simulink model "CH7_4C"  (R2021b)
settings: Solver=ode45  StartTime=0.0  StopTime=4  RelTol=1e-3  EnableMultiTasking=on
libraries: dsparch4 x2
settings Model: Creator=xnote  LastModifiedBy=82102
settings SolverCC: AlgebraicLoopSolver=TrustRegion
settings DataIOCC: LimitDataPoints=on  SaveFormat=Array  SignalLoggingSaveFormat=ModelDataLogs  ReturnWorkspaceOutputs=off
settings OptimizationCC: ExpressionDepthLimit=2147483647  LifeSpan=inf
settings DebuggingCC: UnderspecifiedInitializationDetection=Classic  MergeDetectMultiDrivingBlocksExec=none  SolverPrmCheckMsg=warning  FcnCallInpInsideContextMsg=warning  StateNameClashWarn=warning  SFUnexpectedBacktrackingDiag=warning  SFNoUnconditionalDefaultTransitionDiag=warning  SFExecutionAtInitializationDiag=none  SFMachineParentedDataDiag=warning  ArithmeticOperatorsInVariantConditions=warning
settings HardwareCC: ProdBitPerPointer=32  ProdBitPerSizeT=32  ProdBitPerPtrDiffT=32  ProdLargestAtomicFloat=None  ProdIntDivRoundTo=Undefined  ProdEndianess=Unspecified  ProdWordSize=32  ProdHWDeviceType=32-bit Generic
settings ModelReferenceCC: PropagateSignalLabelsOutOfModel=off
settings SFSimCC: SimUseLocalCustomCode=off  CustomCodeUndefinedFunction=UseInterfaceOnly
settings RTWCC: RTWUseLocalCustomCode=off
settings CodeAppCC: StateflowObjectComments=on
settings GRTTargetCC: TargetLangStandard=C89/C90 (ANSI)  CombineOutputUpdateFcns=off  GRTInterface=on
settings ConfigComp: CovMetricSettings=dw  CovSaveCumulativeToWorkspaceVar=on  CovSaveSingleToWorkspaceVar=on  CovExternalEMLEnable=off

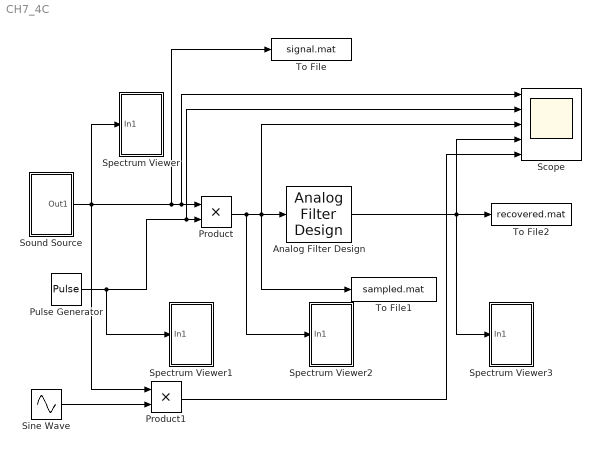
== system CH7_4C ==
  Analog Filter Design : dsparch4/Analog Filter Design  method=Butterworth  filttype=Bandpass  N=8  Wlo=800*pi  Whi=8000*pi  Rp=2  Rs=40
  Product : Product  RndMeth=Zero  SampleTime=1/(16e4)
  Product1 : Product  RndMeth=Zero  SampleTime=1/(16e4)
  Pulse Generator : DiscretePulseGenerator  PulseType=Time based  Period=1/(8e3)  PulseWidth=10
  Scope : Scope  NumInputPorts=5
  Sine Wave : Sin  SampleTime=0
  Sound Source : Subsystem
  Spectrum Viewer : Subsystem
  Spectrum Viewer1 : Subsystem
  Spectrum Viewer2 : Subsystem
  Spectrum Viewer3 : Subsystem
  To File : ToFile  Filename=signal.mat  SampleTime=1/8192
  To File1 : ToFile  Filename=sampled.mat  SampleTime=1/8192
  To File2 : ToFile  Filename=recovered.mat  SampleTime=1/8192
  wires:
  Sound Source/1(Out1) -> Spectrum Viewer/1(In1), To File/1, Product/1, Scope/1, Product1/1
  Pulse Generator/1 -> Spectrum Viewer1/1(In1), Product/2, Scope/2
  Product/1 -> Spectrum Viewer2/1(In1), Analog Filter Design/1, To File1/1, Scope/3
  Analog Filter Design/1 -> To File2/1, Spectrum Viewer3/1(In1), Scope/4
  Sine Wave/1 -> Product1/2
  Product1/1 -> Scope/5

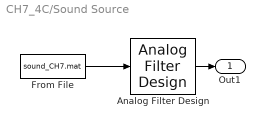
== system CH7_4C/Sound Source ==
  Analog Filter Design : dsparch4/Analog Filter Design  method=Butterworth  filttype=Lowpass  N=8  Wlo=2*pi*4e3  Whi=80  Rp=2  Rs=40
  From File : FromFile  FileName=sound_CH7.mat  SampleTime=0
  Out1 : Outport
  wires:
  From File/1 -> Analog Filter Design/1
  Analog Filter Design/1 -> Out1/1

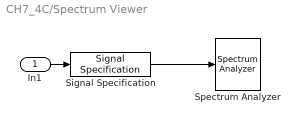
== system CH7_4C/Spectrum Viewer ==
  In1 : Inport
  Signal Specification : SignalSpecification  SampleTime=1/16e4
  Spectrum Analyzer : SpectrumAnalyzer
  wires:
  Signal Specification/1 -> Spectrum Analyzer/1
  In1/1 -> Signal Specification/1

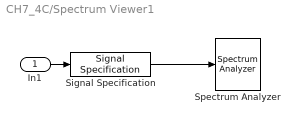
== system CH7_4C/Spectrum Viewer1 ==
  In1 : Inport
  Signal Specification : SignalSpecification  SampleTime=1/16e4
  Spectrum Analyzer : SpectrumAnalyzer
  wires:
  In1/1 -> Signal Specification/1
  Signal Specification/1 -> Spectrum Analyzer/1

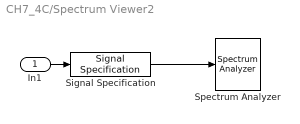
== system CH7_4C/Spectrum Viewer2 ==
  In1 : Inport
  Signal Specification : SignalSpecification  SampleTime=1/16e4
  Spectrum Analyzer : SpectrumAnalyzer
  wires:
  Signal Specification/1 -> Spectrum Analyzer/1
  In1/1 -> Signal Specification/1

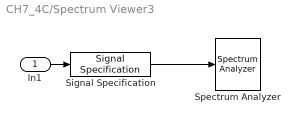
== system CH7_4C/Spectrum Viewer3 ==
  In1 : Inport
  Signal Specification : SignalSpecification  SampleTime=1/16e4
  Spectrum Analyzer : SpectrumAnalyzer
  wires:
  In1/1 -> Signal Specification/1
  Signal Specification/1 -> Spectrum Analyzer/1
